simulink model "ThdRwLtStFwdBkwdHolderChk"  (R2018b)
settings: Solver=FixedStepDiscrete  StartTime=0.0  StopTime=10.0  FixedStep=0.01  RelTol=1e-3
libraries: simulink x2
settings Model: Creator=sn2xws  LastModifiedBy=sn2xws
settings Model: ModifiedHistory=|
  | V2.1.0
  | Bug 547881
  | 干涉信号线未连接导致前后不能动
  | 2024.6.21 V2.2.0 557模式流程V1.6，三排前后需要动2次
  | 25.7.4 V3.13.0 新增Md61 Md62
settings DataIOCC: SaveFormat=StructureWithTime
settings OptimizationCC: DefaultParameterBehavior=Inlined  EnhancedBackFolding=on  PassReuseOutputArgsAs=Individual arguments  ZeroExternalMemoryAtStartup=off  ZeroInternalMemoryAtStartup=off  OptimizeBlockOrder=speed  DifferentSizesBufferReuse=on  OptimizationCustomize=off
settings DebuggingCC: ParameterTunabilityLossMsg=error
settings ModelReferenceCC: ModelReferenceNumInstancesAllowed=Single
settings SFSimCC: MATLABDynamicMemAlloc=off
settings RTWCC: SystemTargetFile=autosar.tlc  GenCodeOnly=on  TemplateMakefile=ert_default_tmf  Description=AUTOSAR  GenerateReport=on  IncludeHyperlinkInReport=on  LaunchReport=on  GenerateTraceInfo=on  GenerateTraceReport=on  GenerateTraceReportSl=on  GenerateTraceReportSf=on  GenerateTraceReportEml=on  GenerateCodeMetricsReport=on
settings CodeAppCC: ForceParamTrailComments=on  IgnoreCustomStorageClasses=off  OperatorAnnotations=on  SimulinkDataObjDesc=on  SFDataObjDesc=on  InsertBlockDesc=on
settings STFCustomTargetCC: TargetLangStandard=C99 (ISO)  MultiwordLength=256  ParMdlRefBuildCompliant=on  CompOptLevelCompliant=on  IncludeMdlTerminateFcn=off  CombineOutputUpdateFcns=on  SuppressErrorStatus=on  ERTCustomFileBanners=on  SupportNonFinite=off  SupportComplex=off  SupportContinuousTime=off  SupportNonInlinedSFcns=off  RemoveResetFunc=on  MATLABClassNameForMDSCustomization=Simulink.SoftwareTarget.ERTCustomization  AutosarCompliant=on  UseToolchainInfoCompliant=on  LookupTableObjectStructAxisOrder=2,1,3,4,...  LUTObjectStructOrderEvenSpacing=Size,Table,Breakpoints  SystemTargetFile=autosar.tlc
settings ERTTargetCC: TargetLangStandard=C99 (ISO)  ConcurrentExecutionCompliant=off  IncludeMdlTerminateFcn=off  SuppressErrorStatus=on  SupportNonFinite=off  SupportComplex=off  ModelStepFunctionPrototypeControlCompliant=off  CPPClassGenCompliant=off  AutosarCompliant=on  LookupTableObjectStructAxisOrder=2,1,3,4,...  LUTObjectStructOrderEvenSpacing=Size,Table,Breakpoints  InlinedParameterPlacement=NonHierarchical  ERTCustomFileTemplate=example_file_process.tlc  ERTFilePackagingFormat=Compact

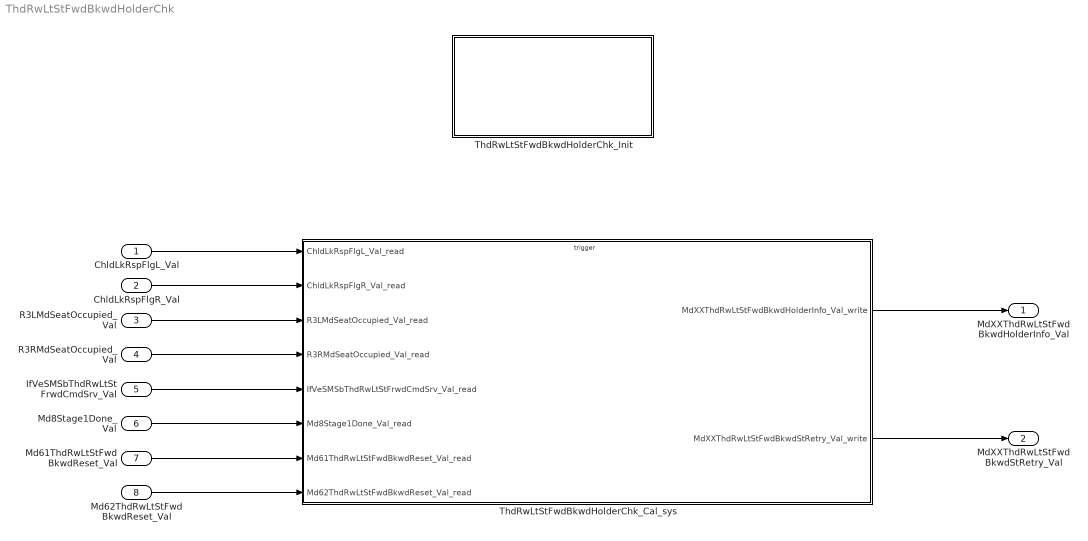
== system ThdRwLtStFwdBkwdHolderChk ==
  ChldLkRspFlgL_Val : Inport  OutDataTypeStr=boolean  PortDimensions=1
  ChldLkRspFlgR_Val : Inport  Port=2  OutDataTypeStr=boolean  PortDimensions=1
  R3LMdSeatOccupied_Val : Inport  Port=3  OutDataTypeStr=boolean  PortDimensions=1
  R3RMdSeatOccupied_Val : Inport  Port=4  OutDataTypeStr=boolean  PortDimensions=1
  IfVeSMSbThdRwLtStFrwdCmdSrv_Val : Inport  Port=5  OutDataTypeStr=boolean  PortDimensions=1
  Md8Stage1Done_Val : Inport  Port=6  OutDataTypeStr=boolean  PortDimensions=1
  Md61ThdRwLtStFwdBkwdReset_Val : Inport  Port=7  OutDataTypeStr=boolean  PortDimensions=1
  Md62ThdRwLtStFwdBkwdReset_Val : Inport  Port=8  OutDataTypeStr=boolean  PortDimensions=1
  ThdRwLtStFwdBkwdHolderChk_Cal_sys : Subsystem
  ThdRwLtStFwdBkwdHolderChk_Init : Subsystem
  MdXXThdRwLtStFwdBkwdHolderInfo_Val : Outport  OutDataTypeStr=uint32  PortDimensions=1
  MdXXThdRwLtStFwdBkwdStRetry_Val : Outport  Port=2  OutDataTypeStr=uint32  PortDimensions=1
  wires:
  ChldLkRspFlgL_Val/1 -> ThdRwLtStFwdBkwdHolderChk_Cal_sys/1(ChldLkRspFlgL_Val_read)
  ChldLkRspFlgR_Val/1 -> ThdRwLtStFwdBkwdHolderChk_Cal_sys/2(ChldLkRspFlgR_Val_read)
  R3LMdSeatOccupied_Val/1 -> ThdRwLtStFwdBkwdHolderChk_Cal_sys/3(R3LMdSeatOccupied_Val_read)
  R3RMdSeatOccupied_Val/1 -> ThdRwLtStFwdBkwdHolderChk_Cal_sys/4(R3RMdSeatOccupied_Val_read)
  ThdRwLtStFwdBkwdHolderChk_Cal_sys/1(MdXXThdRwLtStFwdBkwdHolderInfo_Val_write) -> MdXXThdRwLtStFwdBkwdHolderInfo_Val/1
  IfVeSMSbThdRwLtStFrwdCmdSrv_Val/1 -> ThdRwLtStFwdBkwdHolderChk_Cal_sys/5(IfVeSMSbThdRwLtStFrwdCmdSrv_Val_read)
  Md8Stage1Done_Val/1 -> ThdRwLtStFwdBkwdHolderChk_Cal_sys/6(Md8Stage1Done_Val_read)
  ThdRwLtStFwdBkwdHolderChk_Cal_sys/2(MdXXThdRwLtStFwdBkwdStRetry_Val_write) -> MdXXThdRwLtStFwdBkwdStRetry_Val/1
  Md61ThdRwLtStFwdBkwdReset_Val/1 -> ThdRwLtStFwdBkwdHolderChk_Cal_sys/7(Md61ThdRwLtStFwdBkwdReset_Val_read)
  Md62ThdRwLtStFwdBkwdReset_Val/1 -> ThdRwLtStFwdBkwdHolderChk_Cal_sys/8(Md62ThdRwLtStFwdBkwdReset_Val_read)

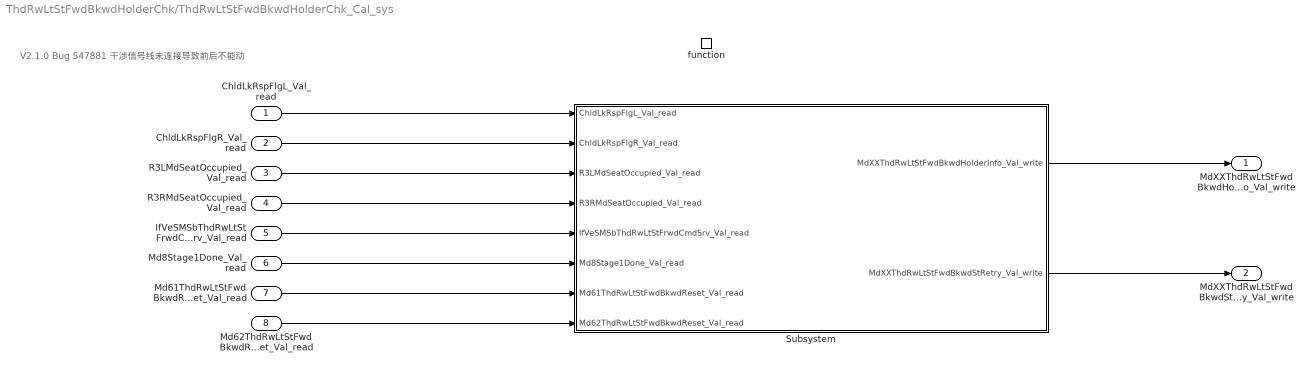
== system ThdRwLtStFwdBkwdHolderChk/ThdRwLtStFwdBkwdHolderChk_Cal_sys ==
  note: V2.1.0
      | Bug 547881 干涉信号线未连接导致前后不能动
  ChldLkRspFlgL_Val_read : Inport
  ChldLkRspFlgR_Val_read : Inport  Port=2
  R3LMdSeatOccupied_Val_read : Inport  Port=3
  R3RMdSeatOccupied_Val_read : Inport  Port=4
  IfVeSMSbThdRwLtStFrwdCmdSrv_Val_read : Inport  Port=5
  Md8Stage1Done_Val_read : Inport  Port=6
  Md61ThdRwLtStFwdBkwdReset_Val_read : Inport  Port=7
  Md62ThdRwLtStFwdBkwdReset_Val_read : Inport  Port=8
  function : TriggerPort  TriggerType=function-call  IsSimulinkFunction=on  FunctionName=ThdRwLtStFwdBkwdHolderChk_Cal  VariantControl=(inherit)
  Subsystem : Subsystem
  MdXXThdRwLtStFwdBkwdHolderInfo_Val_write : Outport
      settings: EnsureOutportIsVirtual=on
  MdXXThdRwLtStFwdBkwdStRetry_Val_write : Outport  Port=2
      settings: EnsureOutportIsVirtual=on
  wires:
  Subsystem/1(MdXXThdRwLtStFwdBkwdHolderInfo_Val_write) -> MdXXThdRwLtStFwdBkwdHolderInfo_Val_write/1
  R3RMdSeatOccupied_Val_read/1 -> Subsystem/4(R3RMdSeatOccupied_Val_read)
  ChldLkRspFlgL_Val_read/1 -> Subsystem/1(ChldLkRspFlgL_Val_read)
  ChldLkRspFlgR_Val_read/1 -> Subsystem/2(ChldLkRspFlgR_Val_read)
  R3LMdSeatOccupied_Val_read/1 -> Subsystem/3(R3LMdSeatOccupied_Val_read)
  IfVeSMSbThdRwLtStFrwdCmdSrv_Val_read/1 -> Subsystem/5(IfVeSMSbThdRwLtStFrwdCmdSrv_Val_read)
  Md8Stage1Done_Val_read/1 -> Subsystem/6(Md8Stage1Done_Val_read)
  Subsystem/2(MdXXThdRwLtStFwdBkwdStRetry_Val_write) -> MdXXThdRwLtStFwdBkwdStRetry_Val_write/1
  Md61ThdRwLtStFwdBkwdReset_Val_read/1 -> Subsystem/7(Md61ThdRwLtStFwdBkwdReset_Val_read)
  Md62ThdRwLtStFwdBkwdReset_Val_read/1 -> Subsystem/8(Md62ThdRwLtStFwdBkwdReset_Val_read)

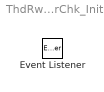
== system ThdRwLtStFwdBkwdHolderChk/ThdRwLtStFwdBkwdHolderChk_Init ==
  Event Listener : EventListener  EventName=reset

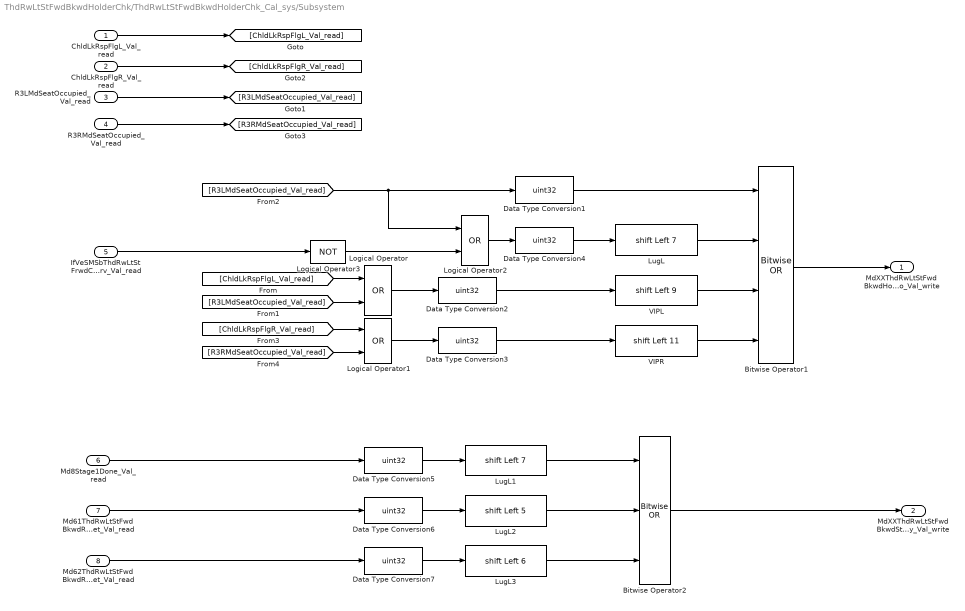
== system ThdRwLtStFwdBkwdHolderChk/ThdRwLtStFwdBkwdHolderChk_Cal_sys/Subsystem ==
  ChldLkRspFlgL_Val_read : Inport
  ChldLkRspFlgR_Val_read : Inport  Port=2
  R3LMdSeatOccupied_Val_read : Inport  Port=3
  R3RMdSeatOccupied_Val_read : Inport  Port=4
  IfVeSMSbThdRwLtStFrwdCmdSrv_Val_read : Inport  Port=5
  Md8Stage1Done_Val_read : Inport  Port=6
  Md61ThdRwLtStFwdBkwdReset_Val_read : Inport  Port=7
  Md62ThdRwLtStFwdBkwdReset_Val_read : Inport  Port=8
  Bitwise Operator1 : simulink/Logic and Bit Operations/Bitwise Operator  logicop=OR  UseBitMask=off  NumInputPorts=4  BitMask=bin2dec('11011001')  BitMaskRealWorld=Stored Integer
  Bitwise Operator2 : simulink/Logic and Bit Operations/Bitwise Operator  logicop=OR  UseBitMask=off  NumInputPorts=3  BitMask=bin2dec('11011001')  BitMaskRealWorld=Stored Integer
  Data Type Conversion{1..7} (7 alike) : DataTypeConversion  OutDataTypeStr=uint32
  Logical Operator : Logic  Operator=OR  AllPortsSameDT=off  OutDataTypeStr=boolean
  Logical Operator1 : Logic  Operator=OR  AllPortsSameDT=off  OutDataTypeStr=boolean
  Logical Operator2 : Logic  Operator=OR  AllPortsSameDT=off  OutDataTypeStr=boolean
  Logical Operator3 : Logic  Operator=NOT  AllPortsSameDT=off  OutDataTypeStr=boolean
  LugL : ArithShift  BitShiftNumber=7  BitShiftDirection=Left
  LugL1 : ArithShift  BitShiftNumber=7  BitShiftDirection=Left
  LugL2 : ArithShift  BitShiftNumber=5  BitShiftDirection=Left
  LugL3 : ArithShift  BitShiftNumber=6  BitShiftDirection=Left
  VIPL : ArithShift  BitShiftNumber=9  BitShiftDirection=Left
  VIPR : ArithShift  BitShiftNumber=11  BitShiftDirection=Left
  MdXXThdRwLtStFwdBkwdHolderInfo_Val_write : Outport
      settings: EnsureOutportIsVirtual=on
  MdXXThdRwLtStFwdBkwdStRetry_Val_write : Outport  Port=2
      settings: EnsureOutportIsVirtual=on
  wires:
  R3RMdSeatOccupied_Val_read/1 -> [R3RMdSeatOccupied_Val_read]
  ChldLkRspFlgL_Val_read/1 -> [ChldLkRspFlgL_Val_read]
  ChldLkRspFlgR_Val_read/1 -> [ChldLkRspFlgR_Val_read]
  R3LMdSeatOccupied_Val_read/1 -> [R3LMdSeatOccupied_Val_read]
  VIPL/1 -> Bitwise Operator1/3
  Data Type Conversion2/1 -> VIPL/1
  Logical Operator/1 -> Data Type Conversion2/1
  [R3RMdSeatOccupied_Val_read] -> Logical Operator1/2
  [R3LMdSeatOccupied_Val_read] -> Logical Operator/2
  Data Type Conversion3/1 -> VIPR/1
  Bitwise Operator1/1 -> MdXXThdRwLtStFwdBkwdHolderInfo_Val_write/1
  LugL/1 -> Bitwise Operator1/2
  [ChldLkRspFlgR_Val_read] -> Logical Operator1/1
  VIPR/1 -> Bitwise Operator1/4
  [ChldLkRspFlgL_Val_read] -> Logical Operator/1
  Logical Operator1/1 -> Data Type Conversion3/1
  [R3LMdSeatOccupied_Val_read] -> Logical Operator2/1, Data Type Conversion1/1
  Data Type Conversion1/1 -> Bitwise Operator1/1
  Logical Operator2/1 -> Data Type Conversion4/1
  IfVeSMSbThdRwLtStFrwdCmdSrv_Val_read/1 -> Logical Operator3/1
  Logical Operator3/1 -> Logical Operator2/2
  Data Type Conversion4/1 -> LugL/1
  Data Type Conversion5/1 -> LugL1/1
  Md8Stage1Done_Val_read/1 -> Data Type Conversion5/1
  LugL1/1 -> Bitwise Operator2/1
  Bitwise Operator2/1 -> MdXXThdRwLtStFwdBkwdStRetry_Val_write/1
  LugL2/1 -> Bitwise Operator2/2
  Md61ThdRwLtStFwdBkwdReset_Val_read/1 -> Data Type Conversion6/1
  Data Type Conversion6/1 -> LugL2/1
  Data Type Conversion7/1 -> LugL3/1
  LugL3/1 -> Bitwise Operator2/3
  Md62ThdRwLtStFwdBkwdReset_Val_read/1 -> Data Type Conversion7/1
